simulink library "odqblock"  (Simulink 7.6)
settings: Solver=ode45  StartTime=0.0  StopTime=10.0  RelTol=1e-3
undefined symbols (not defined in the file or in its folder): d, Ts, x0
settings Model: Creator=morita  LastModifiedBy=moritalocal

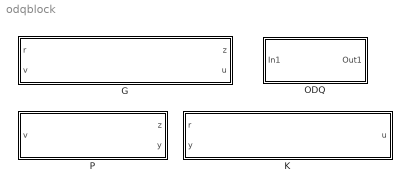
== system odqblock ==
  G : Subsystem  mask(System G){A=0, B1=0, B2=0, C1=0, C2=0, D1=0, D2=0, Ts=Ts, x0=x0}
      mask prompts: Ts "Ts (Sampling Time)"; x0 "Initial Conditions"
      mask help:
      | x(k+1) = A*x(k) + B1*r(k) + B2*v(k)
      |  z(k)  = C1*x(k) + D1*r(k)
      |  u(k)  = C2*x(k) + D2*r(k)
      mask Display:
      | fprintf('%s\n%s\n%s',...
      |     'x[k+1]=A*x[k]+B1*r[k]+B2*v[k]',...
      |     'z[k]=C1*x[k]+D1*r[k]',...
      |     'u[k]=C2*x[k]+D2*r[k]')
      | port_label('input' ,1,'r')
      | port_label('input' ,2,'v')
      | port_label('output',1,'z')
      | port_label('output',2,'u')
  K : Subsystem  mask(Controller K){A=0, B1=0, B2=0, C=0, D1=0, D2=0, Ts=Ts, x0=x0}
      mask prompts: Ts "Ts (Sampling Time)"; x0 "Initial Conditions"
      mask help:
      | x(k+1) = A*x(k) + B1*r(k) + B2*y(k)
      |  u(k)  = C*x(k) + D1*r(k) + D2*y(k)
      mask Display:
      | fprintf('%s\n%s','x[k+1]=A*x[k]+B1*r[k]+B2*y[k]',...
      |     'u[k]=C*x[k]+D1*r[k]+D2*y[k]')
      | port_label('input' ,1,'r')
      | port_label('input' ,2,'y')
      | port_label('output',1,'u')
  ODQ : Subsystem  mask(Opitimal Dynamic Quantizer){A=0, B1=0, B2=0, C=0, d=d, Ts=Ts}
      mask prompts: d "d (Quantization Interval)"; Ts "Ts (Sampling Time)"
      mask help:
      | xi(k+1) = A*xi(k) + B1*u(k) + B2*v(k)
      |   v(k)  = q*[ C*xi(k) + u(k) ]
      mask Help: Please read README.TXT
      mask Display:
      | fprintf('%s','Optimal\nDynamic\nQuantizer')
      | port_label('input' ,1,'u')
      | port_label('output',1,'v')
  P : Subsystem  mask(Plant P){A=0, B=0, C1=0, C2=0, Ts=Ts, x0=x0}
      mask prompts: Ts "Ts (Sampling Time)"; x0 "Initial Conditions"
      mask help:
      | x(k+1) = A*x(k) + B*v(k)
      |  z(k)  = C1*x(k)
      |  y(k)  = C2*x(k)
      mask Display:
      | fprintf('%s\n%s\n%s','x[k+1]=A*x[k]+B*v[k]',...
      |     'z[k]=C1*x[k]',...
      |     'y[k]=C2*x[k]')
      | port_label('input' ,1,'v')
      | port_label('output',1,'z')
      | port_label('output',2,'y')

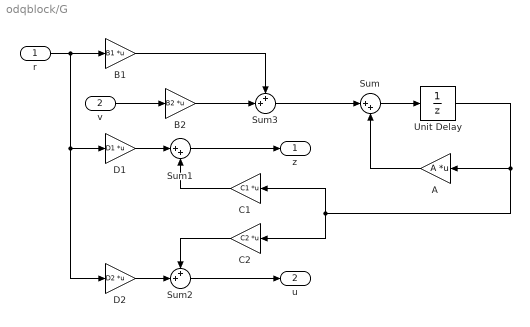
== system odqblock/G ==
  r : Inport
  v : Inport  Port=2
  A : Gain  Gain=A  Multiplication=Matrix(K*u)  SampleTime=Ts
  B1 : Gain  Gain=B1  Multiplication=Matrix(K*u)  SampleTime=Ts
  B2 : Gain  Gain=B2  Multiplication=Matrix(K*u)  SampleTime=Ts
  C1 : Gain  Gain=C1  Multiplication=Matrix(K*u)  SampleTime=Ts
  C2 : Gain  Gain=C2  Multiplication=Matrix(K*u)  SampleTime=Ts
  D1 : Gain  Gain=D1  Multiplication=Matrix(K*u)  SampleTime=Ts
  D2 : Gain  Gain=D2  Multiplication=Matrix(K*u)  SampleTime=Ts
  Sum : Sum  Inputs=|++
  Sum1 : Sum  Inputs=|++
  Sum2 : Sum  Inputs=++|
  Sum3 : Sum  Inputs=++|
  Unit Delay : UnitDelay  X0=x0  SampleTime=Ts
  z : Outport
  u : Outport  Port=2
  wires:
  A/1 -> Sum/2
  r/1 -> B1/1, D1/1, D2/1
  v/1 -> B2/1
  Sum/1 -> Unit Delay/1
  Unit Delay/1 -> C1/1, C2/1, A/1
  D1/1 -> Sum1/1
  C1/1 -> Sum1/2
  Sum1/1 -> z/1
  Sum2/1 -> u/1
  D2/1 -> Sum2/2
  C2/1 -> Sum2/1
  B2/1 -> Sum3/2
  B1/1 -> Sum3/1
  Sum3/1 -> Sum/1

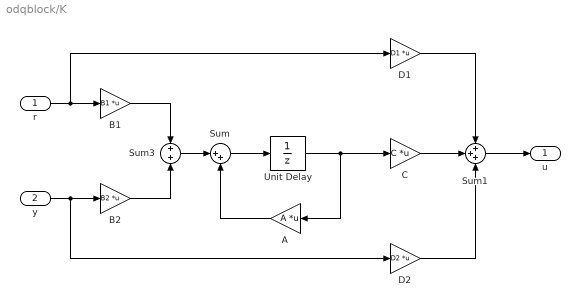
== system odqblock/K ==
  r : Inport
  y : Inport  Port=2
  A : Gain  Gain=A  Multiplication=Matrix(K*u)  SampleTime=Ts
  B1 : Gain  Gain=B1  Multiplication=Matrix(K*u)  SampleTime=Ts
  B2 : Gain  Gain=B2  Multiplication=Matrix(K*u)  SampleTime=Ts
  C : Gain  Gain=C  Multiplication=Matrix(K*u)  SampleTime=Ts
  D1 : Gain  Gain=D1  Multiplication=Matrix(K*u)  SampleTime=Ts
  D2 : Gain  Gain=D2  Multiplication=Matrix(K*u)  SampleTime=Ts
  Sum : Sum  Inputs=|++
  Sum1 : Sum  Inputs=+++
  Sum3 : Sum  Inputs=+|+
  Unit Delay : UnitDelay  X0=x0  SampleTime=Ts
  u : Outport
  wires:
  Sum3/1 -> Sum/1
  B1/1 -> Sum3/1
  B2/1 -> Sum3/2
  Sum1/1 -> u/1
  Unit Delay/1 -> A/1, C/1
  Sum/1 -> Unit Delay/1
  y/1 -> B2/1, D2/1
  r/1 -> B1/1, D1/1
  A/1 -> Sum/2
  C/1 -> Sum1/2
  D2/1 -> Sum1/3
  D1/1 -> Sum1/1

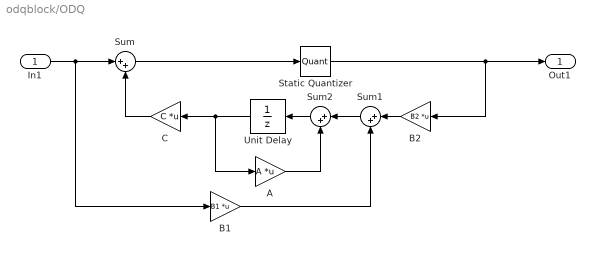
== system odqblock/ODQ ==
  In1 : Inport
  A : Gain  Gain=A  Multiplication=Matrix(K*u)  SampleTime=Ts
  B1 : Gain  Gain=B1  Multiplication=Matrix(K*u)  SampleTime=Ts
  B2 : Gain  Gain=B2  Multiplication=Matrix(K*u)  SampleTime=Ts
  C : Gain  Gain=C  Multiplication=Matrix(K*u)  SampleTime=Ts
  Static Quantizer : Quantizer  QuantizationInterval=d  SampleTime=Ts
  Sum : Sum  Inputs=|++
  Sum1 : Sum  Inputs=|++
  Sum2 : Sum  Inputs=|++
  Unit Delay : UnitDelay  SampleTime=Ts
  Out1 : Outport
  wires:
  In1/1 -> Sum/1, B1/1
  Sum2/1 -> Unit Delay/1
  A/1 -> Sum2/2
  Sum1/1 -> Sum2/1
  B1/1 -> Sum1/2
  B2/1 -> Sum1/1
  Unit Delay/1 -> C/1, A/1
  Static Quantizer/1 -> Out1/1, B2/1
  Sum/1 -> Static Quantizer/1
  C/1 -> Sum/2

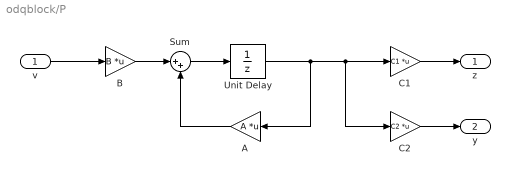
== system odqblock/P ==
  v : Inport
  A : Gain  Gain=A  Multiplication=Matrix(K*u)  SampleTime=Ts
  B : Gain  Gain=B  Multiplication=Matrix(K*u)  SampleTime=Ts
  C1 : Gain  Gain=C1  Multiplication=Matrix(K*u)  SampleTime=Ts
  C2 : Gain  Gain=C2  Multiplication=Matrix(K*u)  SampleTime=Ts
  Sum : Sum  Inputs=|++
  Unit Delay : UnitDelay  X0=x0  SampleTime=Ts
  z : Outport
  y : Outport  Port=2
  wires:
  B/1 -> Sum/1
  C2/1 -> y/1
  C1/1 -> z/1
  Unit Delay/1 -> A/1, C2/1, C1/1
  Sum/1 -> Unit Delay/1
  v/1 -> B/1
  A/1 -> Sum/2
